simulink model "LV"  (Simulink 9.2)
settings: Solver=VariableStepAuto  StartTime=0.0  StopTime=60  MaxStep=1e-4  RelTol=1e-6
settings Model: Creator=jinwooro  LastModifiedBy=jinwooro
settings DataIOCC: LimitDataPoints=off  SaveFormat=Dataset  SignalLoggingSaveFormat=Dataset
settings OptimizationCC: LifeSpan=auto
settings DebuggingCC: UnderspecifiedInitializationDetection=Simplified  MergeDetectMultiDrivingBlocksExec=error  FcnCallInpInsideContextMsg=error  StateNameClashWarn=none  SFUnexpectedBacktrackingDiag=error  SFNoUnconditionalDefaultTransitionDiag=error  SFExecutionAtInitializationDiag=warning
settings HardwareCC: ProdBitPerPointer=64  ProdBitPerSizeT=64  ProdBitPerPtrDiffT=64  ProdLargestAtomicFloat=Float  ProdIntDivRoundTo=Zero  ProdEndianess=LittleEndian  ProdWordSize=64  ProdHWDeviceType=Intel->x86-64 (Windows64)
settings ModelReferenceCC: PropagateSignalLabelsOutOfModel=on
settings SFSimCC: SimUseLocalCustomCode=on
settings RTWCC: RTWUseLocalCustomCode=on
settings CodeAppCC: StateflowObjectComments=off
settings GRTTargetCC: TargetLangStandard=C99 (ISO)  GeneratePreprocessorConditionals=Use local settings  CombineOutputUpdateFcns=on  GRTInterface=off
settings ConfigComp: CovMetricSettings=dwe  CovHtmlReporting=off  CovSaveCumulativeToWorkspaceVar=off  CovSaveSingleToWorkspaceVar=off  CovExternalEMLEnable=on

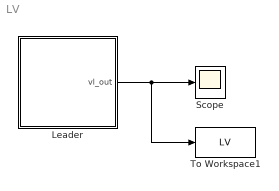
== system LV ==
  Leader : Stateflow chart  TreatAsAtomicUnit=on
  Scope : Scope
  To Workspace1 : ToWorkspace  VariableName=LV  SaveFormat=Timeseries  SampleTime=-1
  wires:
  Leader/1(vl_out) -> To Workspace1/1, Scope/1

== stateflow chart Leader ==
  settings: updateMethod=CONTINUOUS
  state ConstAcc
    du:
    vl_dot = -3 * cos(3 * pi * tau) + 3;
    tau_dot = 0;
    vl_out = vl;
  state IncAcc
    du:
    vl_dot = -3 * cos(3 *pi * tau) + 3;
    tau_dot = 1;
    vl_out = vl;
  state DecAcc
    du:
    vl_dot = - 0.7 * vl * (1 - vl / 17) - 0.2;
    tau_dot = 0;
    vl_out = vl;
  IncAcc -> ConstAcc : [-cos(3 * pi * tau) >= 0.999]
  ConstAcc -> DecAcc : [vl >= 17]
  (default) -> DecAcc : {vl = 17;
      | tau = 0;}
  DecAcc -> IncAcc : [vl <= 0 ]{tau = 0;}
  data: vl local double; vl_out output double; tau local double
  data vl settings: updateMethod=SF_CONTINUOUS_TIME_DATA
  data tau settings: updateMethod=SF_CONTINUOUS_TIME_DATA
